simulink model "ADRC_sim"  (R2023b)
settings: Solver=ode1  StartTime=0.0  StopTime=2  FixedStep=0.001  RelTol=1e-3
settings Model: Creator=Y  LastModifiedBy=Y

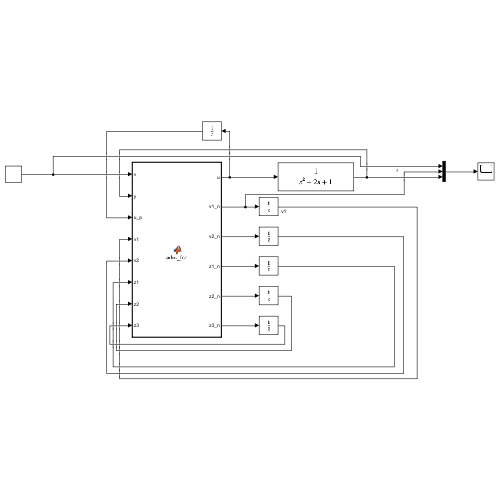
[thumbnail: Simulink's stored preview of the top-level diagram]
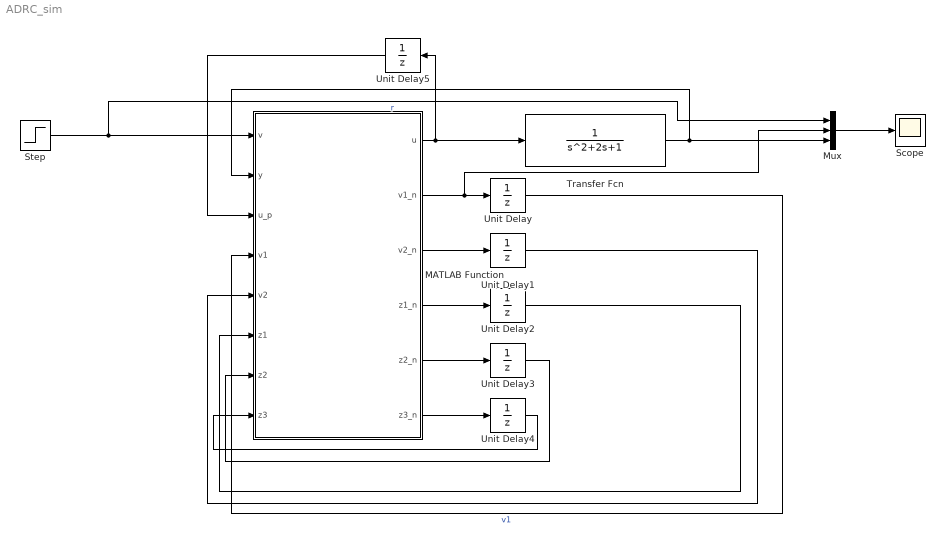
== system ADRC_sim ==
  MATLAB Function : MATLAB Function  TreatAsAtomicUnit=on
  Mux : Mux  Inputs=3
  Scope : Scope
  Step : Step  SampleTime=0
  Transfer Fcn : TransferFcn
  Unit Delay{,1..5} (6 alike) : UnitDelay  SampleTime=-1  HasFrameUpgradeWarning=on
  wires:
  MATLAB Function/6(z3_n) -> Unit Delay4/1
  MATLAB Function/5(z2_n) -> Unit Delay3/1
  MATLAB Function/4(z1_n) -> Unit Delay2/1
  MATLAB Function/3(v2_n) -> Unit Delay1/1
  MATLAB Function/2(v1_n) -> Mux/2, Unit Delay/1
  Step/1 -> Mux/1, MATLAB Function/1(v)  "r"
  MATLAB Function/1(u) -> Unit Delay5/1, Transfer Fcn/1
  Transfer Fcn/1 -> Mux/3, MATLAB Function/2(y)
  Unit Delay/1 -> MATLAB Function/4(v1)  "v1"
  Unit Delay1/1 -> MATLAB Function/5(v2)
  Unit Delay2/1 -> MATLAB Function/6(z1)
  Unit Delay3/1 -> MATLAB Function/7(z2)
  Unit Delay4/1 -> MATLAB Function/8(z3)
  Unit Delay5/1 -> MATLAB Function/3(u_p)
  Mux/1 -> Scope/1

== matlab function ADRC_sim/MATLAB Function ==
  data: v input; u output; y input; u_p input; v1 input; v2 input; z1 input; z2 input; z3 input; v1_n output; v2_n output; z1_n output; z2_n output; z3_n output
function [u, v1_n, v2_n, z1_n, z2_n, z3_n] = adrc_fcn(v, y, u_p, v1, v2, z1, z2, z3)

h_val = 0.001;
params = struct('h', h_val, 'r0', 100, 'r', 100, 'c', 1, 'h1', 0.004, ...
    'b0', 1, 'beta01', 1, ...
    'beta02', 1/(2*h_val^0.5), ...
    'beta03', 2/(25*h_val^1.2));

[u, v1_n, v2_n, z1_n, z2_n, z3_n] = ...
    adrc_controller(v, y, u_p, v1, v2, z1, z2, z3, params);
end
